simulink model "Amp_baseline_Excel"  (R2020a)
settings: Solver=VariableStepAuto  StartTime=0.0  StopTime=60  RelTol=1e-3
model workspace (MAT data in the model file):
  WinSize = Simulink.Parameter
  WinSize.Value = 16
  WinSize.DataType = 'double'
  WinSize.Dimensions = [1 1]
  fc_bandpass = Simulink.Parameter
  fc_bandpass.Value = [0.05 0.26]
  fc_bandpass.DataType = 'double'
  fc_bandpass.Dimensions = [1 2]
undefined symbols (not defined in the file or in its folder): A1, A138674, I1, J138674
settings Model: Creator=LAB-OREN3  LastModifiedBy=LAB-OREN1

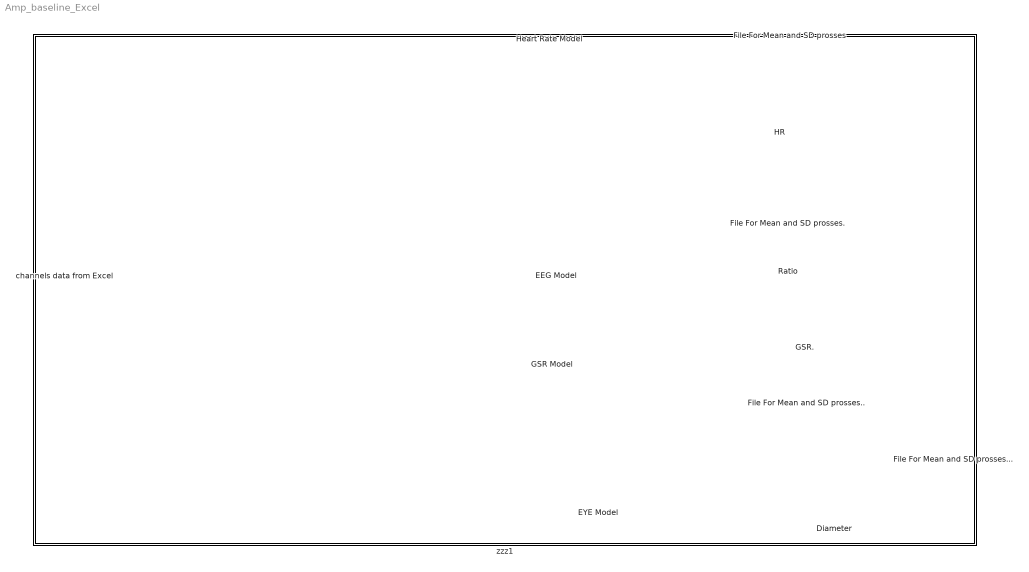
== system Amp_baseline_Excel ==
  Diameter : Display
  EEG Model : Subsystem  ReferencedSubsystem=EEG_Ratio_Model
  EYE Model : Subsystem  ReferencedSubsystem=Pupil_Diameter_Model_BaseLine
  File For Mean and SD prosses : ToFile  Filename=Heartrate.mat  MatrixName=heartRatedata
  File For Mean and SD prosses. : ToFile  Filename=Ratio.mat  MatrixName=Ratio
  File For Mean and SD prosses.. : ToFile  Filename=GSR.mat  MatrixName=GSR
  File For Mean and SD prosses... : ToFile  Filename=Eye_Diameter.mat  MatrixName=Eye_Diameter
  GSR Model : Subsystem
  GSR. : Display
  HR : Display
  Heart Rate Model : Subsystem  ReferencedSubsystem=Heart_Rate_Model
  Ratio : Display
  channels data from Excel : Subsystem
  zzz1 : Subsystem  TreatAsAtomicUnit=on
      settings: OpenFcn=% no-op
      mask Display: disp('')
  wires:
  Heart Rate Model/1 -> File For Mean and SD prosses/1
  GSR Model/1(GSR) -> File For Mean and SD prosses../1, GSR./1
  Heart Rate Model/2 -> HR/1
  EYE Model/1 -> File For Mean and SD prosses.../1, Diameter/1
  EEG Model/1 -> Ratio/1, File For Mean and SD prosses./1
  channels data from Excel/1(ECG) -> Heart Rate Model/1
  channels data from Excel/2(EEG1) -> EEG Model/1
  channels data from Excel/3(EEG2) -> EEG Model/2
  channels data from Excel/4(EEG3) -> EEG Model/3
  channels data from Excel/5(EEG4) -> EEG Model/4
  channels data from Excel/6(EEG5) -> EEG Model/5
  channels data from Excel/7(EEG6) -> EEG Model/6
  channels data from Excel/8(EEG7) -> EEG Model/7
  channels data from Excel/9(EEG8) -> EEG Model/8
  channels data from Excel/10(EEG9) -> EEG Model/9
  channels data from Excel/11(EEG10) -> EEG Model/10
  channels data from Excel/12(EEG11) -> EEG Model/11
  channels data from Excel/13(GSR) -> GSR Model/1(GSR.)
  channels data from Excel/14(Pupil diameter Right) -> EYE Model/1
  channels data from Excel/15(Pupil diameter Left) -> EYE Model/2
  channels data from Excel/16(EEG12) -> EEG Model/12

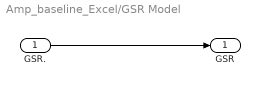
== system Amp_baseline_Excel/GSR Model ==
  GSR. : Inport
  GSR : Outport
  wires:
  GSR./1 -> GSR/1

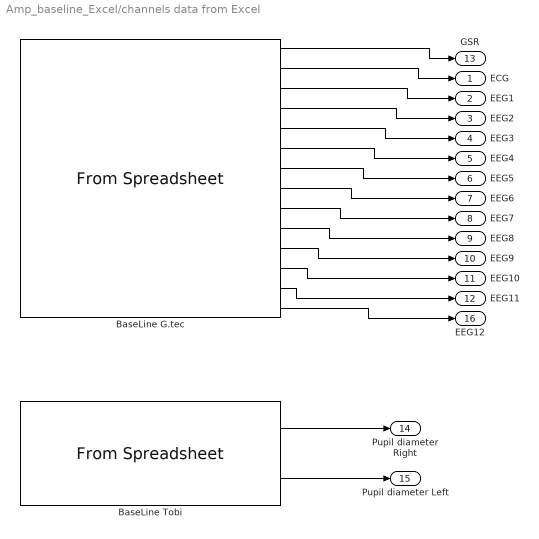
== system Amp_baseline_Excel/channels data from Excel ==
  BaseLine G.tec : FromSpreadsheet  FileName=C:\Users\LAB-OREN1\Downloads\No_Stress.xlsx  SheetName=גיליון1  Range=A1:O30722  SampleTime=0.001953125
  BaseLine Tobi : FromSpreadsheet  FileName=C:\Users\LAB-OREN1\Downloads\Tobii Data of A5_502459_COMBINED_CUBE_DELAY_150_TTC_15 at (13;43;12).xlsx  SheetName=גיליון1  Range=A1:A138674,I1:J138674  SampleTime=0.001953125
  ECG : Outport
  EEG1 : Outport  Port=2
  EEG2 : Outport  Port=3
  EEG3 : Outport  Port=4
  EEG4 : Outport  Port=5
  EEG5 : Outport  Port=6
  EEG6 : Outport  Port=7
  EEG7 : Outport  Port=8
  EEG8 : Outport  Port=9
  EEG9 : Outport  Port=10
  EEG10 : Outport  Port=11
  EEG11 : Outport  Port=12
  GSR : Outport  Port=13
  Pupil diameter Right : Outport  Port=14
  Pupil diameter Left : Outport  Port=15
  EEG12 : Outport  Port=16
  wires:
  BaseLine G.tec/2 -> ECG/1
  BaseLine G.tec/8 -> EEG6/1
  BaseLine G.tec/13 -> EEG11/1
  BaseLine Tobi/1 -> Pupil diameter Right/1
  BaseLine G.tec/4 -> EEG2/1
  BaseLine G.tec/10 -> EEG8/1
  BaseLine G.tec/6 -> EEG4/1
  BaseLine G.tec/12 -> EEG10/1
  BaseLine G.tec/3 -> EEG1/1
  BaseLine G.tec/11 -> EEG9/1
  BaseLine G.tec/9 -> EEG7/1
  BaseLine G.tec/7 -> EEG5/1
  BaseLine G.tec/5 -> EEG3/1
  BaseLine Tobi/2 -> Pupil diameter Left/1
  BaseLine G.tec/1 -> GSR/1
  BaseLine G.tec/14 -> EEG12/1

== system Amp_baseline_Excel/zzz1 ==
